simulink model "PID_Controller"  (R2020b)
settings: Solver=VariableStepAuto  StartTime=0.0  StopTime=10.0  RelTol=1e-3
PreLoadFcn:
  | kd = -0.0152524604;
  | ki = 0.087984779779;
  | kp = 0.669524552;
settings Model: Creator=sai  LastModifiedBy=sai

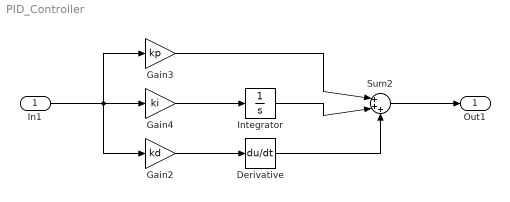
== system PID_Controller ==
  In1 : Inport  OutDataTypeStr=double  PortDimensions=1  SampleTime=0
  Derivative : Derivative
  Gain2 : Gain  Gain=kd
  Gain3 : Gain  Gain=kp
  Gain4 : Gain  Gain=ki
  Integrator : Integrator
  Sum2 : Sum  Inputs=|+++
  Out1 : Outport  OutDataTypeStr=double  PortDimensions=1  SampleTime=0
  wires:
  Gain4/1 -> Integrator/1
  Gain3/1 -> Sum2/1
  In1/1 -> Gain4/1, Gain3/1, Gain2/1
  Derivative/1 -> Sum2/3
  Integrator/1 -> Sum2/2
  Gain2/1 -> Derivative/1
  Sum2/1 -> Out1/1
